simulink model "DC_Motor_Puls"  (R2018a)
settings: Solver=ode45  StartTime=0.0  StopTime=0.2  MaxStep=0.0000008  RelTol=1e-8  EnableMultiTasking=on
values from neighbouring files (symbols this model uses):
  J_ges = 54e-6    (= 5.4e-05)    [bldc_motor.m]    (also in test_DC_Motor.m = 1.07037741047e-06)
  La = 10*1.792e-3    (= 0.01792)    [test_DC_Motor.m]
  M_motor = I_out*Psi    [test_DC_Motor.m]
  Mo = Io*Psi    (= 0.00055809)    [test_DC_Motor.m]
  Psi = 0.0265    [bldc_motor.m]    (also in test_DC_Motor.m = 0.0159)
  Ra = 6.7    [test_DC_Motor.m]
  T_on = 0.003    [test_DC_Motor.m]
  U_max = 8    [test_DC_Motor.m]
settings Model: Creator=dep02378  LastModifiedBy=Horst
settings DataIOCC: LimitDataPoints=on  SaveFormat=Array  SignalLoggingSaveFormat=ModelDataLogs
settings OptimizationCC: ExpressionDepthLimit=2147483647  InitFltsAndDblsToZero=on  LifeSpan=inf
settings DebuggingCC: UnderspecifiedInitializationDetection=Classic  MergeDetectMultiDrivingBlocksExec=none  SolverPrmCheckMsg=warning  FcnCallInpInsideContextMsg=warning  StateNameClashWarn=warning  SFUnexpectedBacktrackingDiag=warning  SFNoUnconditionalDefaultTransitionDiag=warning  SFExecutionAtInitializationDiag=none
settings HardwareCC: ProdBitPerPointer=32  ProdBitPerSizeT=32  ProdBitPerPtrDiffT=32  ProdLargestAtomicFloat=None  ProdIntDivRoundTo=Undefined  ProdEndianess=Unspecified  ProdWordSize=32  ProdHWDeviceType=32-bit Generic
settings ModelReferenceCC: PropagateSignalLabelsOutOfModel=off
settings CodeAppCC: StateflowObjectComments=on
settings GRTTargetCC: TargetLangStandard=C89/C90 (ANSI)  GeneratePreprocessorConditionals=Disable all  CombineOutputUpdateFcns=off  GRTInterface=on
settings ConfigComp: CovMetricSettings=dw  CovHtmlReporting=on  CovSaveCumulativeToWorkspaceVar=on  CovSaveSingleToWorkspaceVar=on  CovExternalEMLEnable=off

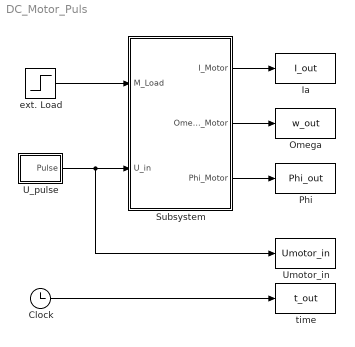
== system DC_Motor_Puls ==
  Clock : Clock
  Ia : ToWorkspace  VariableName=I_out  SampleTime=-1
  Omega : ToWorkspace  VariableName=w_out  SampleTime=-1
  Phi : ToWorkspace  VariableName=Phi_out  SampleTime=-1
  Subsystem : Subsystem
  U_pulse : Subsystem
  Umotor_in : ToWorkspace  VariableName=Umotor_in  SampleTime=-1
  ext. Load : Step  Time=0  After=M_motor  SampleTime=0
  time : ToWorkspace  VariableName=t_out  SampleTime=-1
  wires:
  Clock/1 -> time/1
  ext. Load/1 -> Subsystem/1(M_Load)
  Subsystem/3(Phi_Motor) -> Phi/1
  U_pulse/1(Pulse) -> Umotor_in/1, Subsystem/2(U_in)
  Subsystem/1(I_Motor) -> Ia/1
  Subsystem/2(Omega_Motor) -> Omega/1

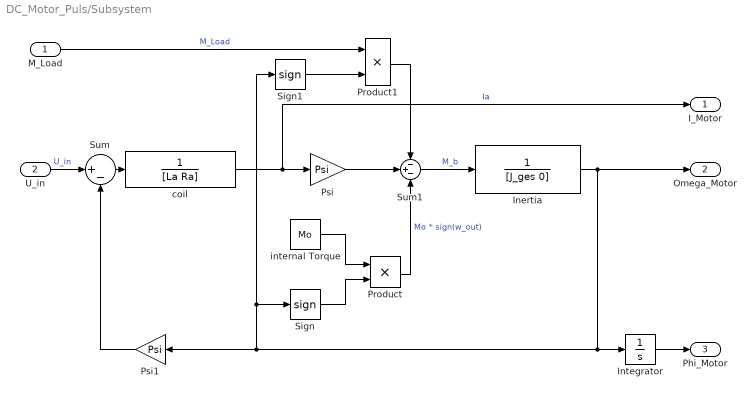
== system DC_Motor_Puls/Subsystem ==
  M_Load : Inport
  U_in : Inport  Port=2
  Inertia : TransferFcn  Denominator=[J_ges 0]
  Integrator : Integrator
  Product : Product  RndMeth=Zero
  Product1 : Product  RndMeth=Zero
  Psi : Gain  Gain=Psi
  Psi1 : Gain  Gain=Psi
  Sign : Signum  ZeroCross=off
  Sign1 : Signum  ZeroCross=off
  Sum : Sum  Inputs=|+-
  Sum1 : Sum  Inputs=-+-
  coil : TransferFcn  Denominator=[La Ra]
  internal Torque : Constant  Value=Mo
  I_Motor : Outport
  Omega_Motor : Outport  Port=2
  Phi_Motor : Outport  Port=3
  wires:
  Sum/1 -> coil/1
  coil/1 -> Psi/1, I_Motor/1  "Ia"
  Inertia/1 -> Psi1/1, Sign/1, Sign1/1, Integrator/1, Omega_Motor/1
  Sum1/1 -> Inertia/1  "M_b"
  Psi/1 -> Sum1/2
  Product/1 -> Sum1/3  "Mo * sign(w_out)"
  internal Torque/1 -> Product/1
  Sign/1 -> Product/2
  Integrator/1 -> Phi_Motor/1
  Product1/1 -> Sum1/1
  Sign1/1 -> Product1/2
  M_Load/1 -> Product1/1  "M_Load"
  U_in/1 -> Sum/1  "U_in"
  Psi1/1 -> Sum/2

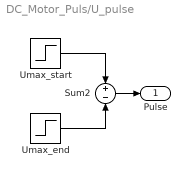
== system DC_Motor_Puls/U_pulse ==
  Sum2 : Sum  Inputs=+-
  Umax_end : Step  Time=T_on  After=U_max  SampleTime=0
  Umax_start : Step  Time=0  Before=T_on  After=U_max  SampleTime=0
  Pulse : Outport
  wires:
  Umax_end/1 -> Sum2/2
  Umax_start/1 -> Sum2/1
  Sum2/1 -> Pulse/1
